simulink model "Fixed_Formation"  (R2014a)
settings: Solver=ode45  StartTime=0.0  StopTime=100.0  RelTol=1e-3
libraries: simulink x4
settings Model: Creator=asus  LastModifiedBy=asus

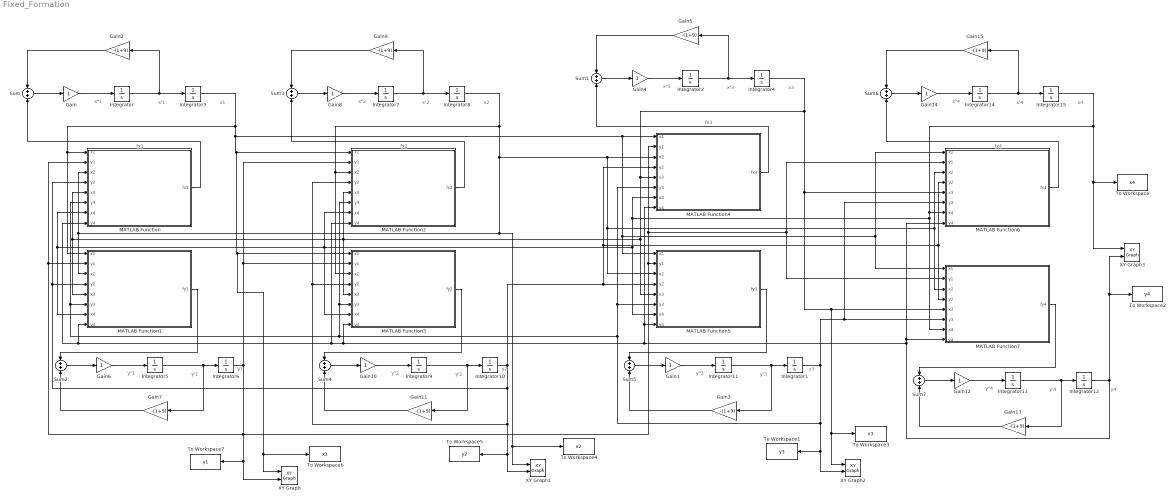
== system Fixed_Formation ==
  note: x1
  note: x'1
  note: x"1
  note: fx1
  note: y1
  note: y'1
  note: y"1
  note: x2
  note: x'2
  note: x"2
  note: fx2
  note: y2
  note: y'2
  note: y"2
  note: x3
  note: x'3
  note: x"3
  note: fx3
  note: y3
  note: y'3
  note: y"3
  note: x4
  note: x'4
  note: x"4
  note: fx4
  note: y4
  note: y'4
  note: y"4
  Gain{,1,4,6,8,10,12,14} (8 alike) : Gain
  Gain{2..3,5,7,9,11,13,15} (8 alike) : Gain  Gain=-(1+9)
  Integrator{,2,5,7,9,11,13..14} (8 alike) : Integrator
  Integrator1 : Integrator  InitialCondition=2
  Integrator10 : Integrator  InitialCondition=1
  Integrator12 : Integrator  InitialCondition=4
  Integrator15 : Integrator  InitialCondition=4
  Integrator3 : Integrator  InitialCondition=-3
  Integrator4 : Integrator  InitialCondition=5
  Integrator6 : Integrator  InitialCondition=3
  Integrator8 : Integrator  InitialCondition=1
  MATLAB Function : MATLAB Function  TreatAsAtomicUnit=on
  MATLAB Function1 : MATLAB Function  TreatAsAtomicUnit=on
  MATLAB Function2 : MATLAB Function  TreatAsAtomicUnit=on
  MATLAB Function3 : MATLAB Function  TreatAsAtomicUnit=on
  MATLAB Function4 : MATLAB Function  TreatAsAtomicUnit=on
  MATLAB Function5 : MATLAB Function  TreatAsAtomicUnit=on
  MATLAB Function6 : MATLAB Function  TreatAsAtomicUnit=on
  MATLAB Function7 : MATLAB Function  TreatAsAtomicUnit=on
  Sum{,1..7} (8 alike) : Sum  Inputs=+|+
  To Workspace : ToWorkspace  VariableName=x4  SampleTime=0.01
  To Workspace1 : ToWorkspace  VariableName=y3  SampleTime=0.01
  To Workspace2 : ToWorkspace  VariableName=y4  SampleTime=0.01
  To Workspace3 : ToWorkspace  VariableName=x3  SampleTime=0.01
  To Workspace4 : ToWorkspace  VariableName=x2  SampleTime=0.01
  To Workspace5 : ToWorkspace  VariableName=y2  SampleTime=0.01
  To Workspace6 : ToWorkspace  VariableName=x1  SampleTime=0.01
  To Workspace7 : ToWorkspace  VariableName=y1  SampleTime=0.01
  XY Graph{,1..3} (4 alike) : simulink/Sinks/XY Graph  xmin=-10  xmax=10  ymin=-10  ymax=10  st=0.01
  wires:
  Sum/1 -> Gain/1
  Gain/1 -> Integrator/1
  Integrator/1 -> Gain2/1, Integrator3/1
  Gain2/1 -> Sum/1
  Integrator3/1 -> MATLAB Function6/1(x1), MATLAB Function7/1(x1), MATLAB Function5/1(x1), MATLAB Function4/1(x1), To Workspace6/1, XY Graph/1, MATLAB Function3/1(x1), MATLAB Function2/1(x1), MATLAB Function/1(x1), MATLAB Function1/1(x1)
  Sum2/1 -> Gain6/1
  Gain6/1 -> Integrator5/1
  Integrator5/1 -> Gain7/1, Integrator6/1
  Gain7/1 -> Sum2/2
  MATLAB Function1/1(fy1) -> Sum2/1
  Sum3/1 -> Gain8/1
  Gain8/1 -> Integrator7/1
  Integrator7/1 -> Gain9/1, Integrator8/1
  Gain9/1 -> Sum3/1
  Integrator8/1 -> MATLAB Function7/3(x2), MATLAB Function6/3(x2), MATLAB Function5/3(x2), MATLAB Function4/3(x2), To Workspace4/1, XY Graph1/1, MATLAB Function1/3(x2), MATLAB Function/3(x2), MATLAB Function3/3(x2), MATLAB Function2/3(x2)
  MATLAB Function2/1(fx2) -> Sum3/2
  Sum4/1 -> Gain10/1
  Gain10/1 -> Integrator9/1
  Integrator9/1 -> Gain11/1, Integrator10/1
  Gain11/1 -> Sum4/2
  MATLAB Function3/1(fy2) -> Sum4/1
  Sum1/1 -> Gain4/1
  Gain4/1 -> Integrator2/1
  Integrator2/1 -> Gain5/1, Integrator4/1
  Gain5/1 -> Sum1/1
  MATLAB Function4/1(fx3) -> Sum1/2
  Sum5/1 -> Gain1/1
  Gain1/1 -> Integrator11/1
  Integrator11/1 -> Gain3/1, Integrator1/1
  Gain3/1 -> Sum5/2
  MATLAB Function5/1(fy3) -> Sum5/1
  Integrator1/1 -> MATLAB Function6/6(y3), MATLAB Function7/6(y3), To Workspace1/1, XY Graph2/2, MATLAB Function/6(y3), MATLAB Function1/6(y3), MATLAB Function3/6(y3), MATLAB Function2/6(y3), MATLAB Function5/6(y3), MATLAB Function4/6(y3)
  Sum6/1 -> Gain14/1
  Gain14/1 -> Integrator14/1
  Integrator14/1 -> Gain15/1, Integrator15/1
  Gain15/1 -> Sum6/1
  Integrator15/1 -> To Workspace/1, XY Graph3/1, MATLAB Function1/7(x4), MATLAB Function/7(x4), MATLAB Function3/7(x4), MATLAB Function2/7(x4), MATLAB Function5/7(x4), MATLAB Function4/7(x4), MATLAB Function7/7(x4), MATLAB Function6/7(x4)
  MATLAB Function6/1(fx4) -> Sum6/2
  Sum7/1 -> Gain12/1
  Gain12/1 -> Integrator13/1
  Integrator13/1 -> Gain13/1, Integrator12/1
  Gain13/1 -> Sum7/2
  MATLAB Function7/1(fy4) -> Sum7/1
  Integrator4/1 -> MATLAB Function6/5(x3), To Workspace3/1, XY Graph2/1, MATLAB Function7/5(x3), MATLAB Function4/5(x3), MATLAB Function5/5(x3), MATLAB Function1/5(x3), MATLAB Function/5(x3), MATLAB Function2/5(x3), MATLAB Function3/5(x3)
  Integrator12/1 -> To Workspace2/1, XY Graph3/2, MATLAB Function6/8(y4), MATLAB Function7/8(y4), MATLAB Function4/8(y4), MATLAB Function5/8(y4), MATLAB Function2/8(y4), MATLAB Function/8(y4), MATLAB Function1/8(y4), MATLAB Function3/8(y4)
  Integrator10/1 -> MATLAB Function6/4(y2), MATLAB Function7/4(y2), MATLAB Function4/4(y2), MATLAB Function5/4(y2), MATLAB Function/4(y2), MATLAB Function1/4(y2), To Workspace5/1, XY Graph1/2, MATLAB Function2/4(y2), MATLAB Function3/4(y2)
  Integrator6/1 -> MATLAB Function2/2(y1), MATLAB Function3/2(y1), To Workspace7/1, XY Graph/2, MATLAB Function7/2(y1), MATLAB Function6/2(y1), MATLAB Function4/2(y1), MATLAB Function5/2(y1), MATLAB Function/2(y1), MATLAB Function1/2(y1)
  MATLAB Function/1(fx1) -> Sum/2

== matlab function Fixed_Formation/MATLAB Function1 ==
  data: fy1 output; x1 input; y1 input; x2 input; y2 input; x3 input; y3 input; x4 input; y4 input
function fy1 = fy1(x1,y1,x2,y2,x3,y3,x4,y4)
%#codegen
% Agent N#1
%xc = sin(t);
%yc = t;

xc = 0;             % X-Center.
yc = 0;             % Y-Center.
al = 3;             % Radius.
x = [x1 x2 x3 x4];      
y = [y1 y2 y3 y4];     
M = 1;              % Mass.
B = 1;              % Damper.
kd = 9;             % Overshoot Controlling Coefficient.
ks = 1;
q = 10;     % Charges.
kr = 0.15;
N = 4;              % Number od Agents.

r2 = zeros(N,N);
costet = zeros(N,N);
sintet = zeros(N,N);
Prx = zeros(N);
Pry = zeros(N);

fx = zeros(N);
fy = zeros(N);
Fx = zeros(N);
Fy = zeros(N);

for k=1:N
    
    for i=1:N
      Pr = 0;
      r2(k,i) = ((x(i)-x(k))^2)+((y(i)-y(k))^2);
    
      if i==k
         Prx(k) = Prx(k) + 0;
         Pry(k) = Pry(k) + 0;
      else
         costet(k,i) = (x(k)-x(i))/sqrt(r2(k,i));
         sintet(k,i) = (y(k)-y(i))/sqrt(r2(k,i));
         Prx(k) = Prx(k) + (q*q/r2(k,i))*costet(k,i);
         Pry(k) = Pry(k) + (q*q/r2(k,i))*sintet(k,i);
        
      end
    end

    Fx(k) = kr*Prx(k);
    Fy(k) = kr*Pry(k);
                        
    fx(k) = Fx(k)-ks*((x(k)-xc)*(((x(k)-xc)^2)+((y(k)-yc)^2)-al^2));
    fy(k) = Fy(k)-ks*((y(k)-yc)*(((x(k)-xc)^2)+((y(k)-yc)^2)-al^2));

end

fy1 = fy(1);

end

== matlab function Fixed_Formation/MATLAB Function ==
  data: fx1 output; x1 input; y1 input; x2 input; y2 input; x3 input; y3 input; x4 input; y4 input
function fx1 = fx1(x1,y1,x2,y2,x3,y3,x4,y4)
%#codegen
% Agent N#1

xc = 0;             % X-Center.
yc = 0;             % Y-Center.
al = 3;             % Radius.
x = [x1 x2 x3 x4];      
y = [y1 y2 y3 y4];     
M = 1;              % Mass.
B = 1;              % Damper.
kd = 9;             % Overshoot Controlling Coefficient.
ks = 1;
q = 10;     % Charges.
kr = 0.15;
N = 4;              % Number od Agents.

r2 = zeros(N,N);
costet = zeros(N,N);
sintet = zeros(N,N);
Prx = zeros(N);
Pry = zeros(N);

fx = zeros(N);
fy = zeros(N);
Fx = zeros(N);
Fy = zeros(N);

for k=1:N
    
    for i=1:N
      Pr = 0;
      r2(k,i) = ((x(i)-x(k))^2)+((y(i)-y(k))^2);
    
      if i==k
         Prx(k) = Prx(k) + 0;
         Pry(k) = Pry(k) + 0;
      else
         costet(k,i) = (x(k)-x(i))/sqrt(r2(k,i));
         sintet(k,i) = (y(k)-y(i))/sqrt(r2(k,i));
         Prx(k) = Prx(k) + (q*q/r2(k,i))*costet(k,i);
         Pry(k) = Pry(k) + (q*q/r2(k,i))*sintet(k,i);
        
      end
    end

    Fx(k) = kr*Prx(k);
    Fy(k) = kr*Pry(k);
                        
    fx(k) = Fx(k)-ks*((x(k)-xc)*(((x(k)-xc)^2)+((y(k)-yc)^2)-al^2));
    fy(k) = Fy(k)-ks*((y(k)-yc)*(((x(k)-xc)^2)+((y(k)-yc)^2)-al^2));

end

fx1 = fx(1);

end

== matlab function Fixed_Formation/MATLAB Function2 ==
  data: fx2 output; x1 input; y1 input; x2 input; y2 input; x3 input; y3 input; x4 input; y4 input
function fx2 = fx2(x1,y1,x2,y2,x3,y3,x4,y4)
%#codegen
% Agent N#1

xc = 0;             % X-Center.
yc = 0;             % Y-Center.
al = 3;             % Radius.
x = [x1 x2 x3 x4];      
y = [y1 y2 y3 y4];     
M = 1;              % Mass.
B = 1;              % Damper.
kd = 9;             % Overshoot Controlling Coefficient.
ks = 1;
q = 10;     % Charges.
kr = 0.15;
N = 4;              % Number od Agents.

r2 = zeros(N,N);
costet = zeros(N,N);
sintet = zeros(N,N);
Prx = zeros(N);
Pry = zeros(N);

fx = zeros(N);
fy = zeros(N);
Fx = zeros(N);
Fy = zeros(N);

for k=1:N
    
    for i=1:N
      Pr = 0;
      r2(k,i) = ((x(i)-x(k))^2)+((y(i)-y(k))^2);
    
      if i==k
         Prx(k) = Prx(k) + 0;
         Pry(k) = Pry(k) + 0;
      else
         costet(k,i) = (x(k)-x(i))/sqrt(r2(k,i));
         sintet(k,i) = (y(k)-y(i))/sqrt(r2(k,i));
         Prx(k) = Prx(k) + (q*q/r2(k,i))*costet(k,i);
         Pry(k) = Pry(k) + (q*q/r2(k,i))*sintet(k,i);
        
      end
    end

    Fx(k) = kr*Prx(k);
    Fy(k) = kr*Pry(k);
                        
    fx(k) = Fx(k)-ks*((x(k)-xc)*(((x(k)-xc)^2)+((y(k)-yc)^2)-al^2));
    fy(k) = Fy(k)-ks*((y(k)-yc)*(((x(k)-xc)^2)+((y(k)-yc)^2)-al^2));

end

fx2 = fx(2);


end

== matlab function Fixed_Formation/MATLAB Function3 ==
  data: fy2 output; x1 input; y1 input; x2 input; y2 input; x3 input; y3 input; x4 input; y4 input
function fy2 = fy2(x1,y1,x2,y2,x3,y3,x4,y4)
%#codegen
% Agent N#1

xc = 0;             % X-Center.
yc = 0;             % Y-Center.
al = 3;             % Radius.
x = [x1 x2 x3 x4];      
y = [y1 y2 y3 y4];     
M = 1;              % Mass.
B = 1;              % Damper.
kd = 9;             % Overshoot Controlling Coefficient.
ks = 1;
q = 10;     % Charges.
kr = 0.15;
N = 4;              % Number od Agents.

r2 = zeros(N,N);
costet = zeros(N,N);
sintet = zeros(N,N);
Prx = zeros(N);
Pry = zeros(N);

fx = zeros(N);
fy = zeros(N);
Fx = zeros(N);
Fy = zeros(N);

for k=1:N
    
    for i=1:N
      Pr = 0;
      r2(k,i) = ((x(i)-x(k))^2)+((y(i)-y(k))^2);
    
      if i==k
         Prx(k) = Prx(k) + 0;
         Pry(k) = Pry(k) + 0;
      else
         costet(k,i) = (x(k)-x(i))/sqrt(r2(k,i));
         sintet(k,i) = (y(k)-y(i))/sqrt(r2(k,i));
         Prx(k) = Prx(k) + (q*q/r2(k,i))*costet(k,i);
         Pry(k) = Pry(k) + (q*q/r2(k,i))*sintet(k,i);
        
      end
    end

    Fx(k) = kr*Prx(k);
    Fy(k) = kr*Pry(k);
                        
    fx(k) = Fx(k)-ks*((x(k)-xc)*(((x(k)-xc)^2)+((y(k)-yc)^2)-al^2));
    fy(k) = Fy(k)-ks*((y(k)-yc)*(((x(k)-xc)^2)+((y(k)-yc)^2)-al^2));

end

fy2 = fy(2);


end

== matlab function Fixed_Formation/MATLAB Function4 ==
  data: fx3 output; x1 input; y1 input; x2 input; y2 input; x3 input; y3 input; x4 input; y4 input
function fx3 = fx3(x1,y1,x2,y2,x3,y3,x4,y4)
%#codegen
% Agent N#1

xc = 0;             % X-Center.
yc = 0;             % Y-Center.
al = 3;             % Radius.
x = [x1 x2 x3 x4];      
y = [y1 y2 y3 y4];     
M = 1;              % Mass.
B = 1;              % Damper.
kd = 9;             % Overshoot Controlling Coefficient.
ks = 1;
q = 10;     % Charges.
kr = 0.15;
N = 4;              % Number od Agents.

r2 = zeros(N,N);
costet = zeros(N,N);
sintet = zeros(N,N);
Prx = zeros(N);
Pry = zeros(N);

fx = zeros(N);
fy = zeros(N);
Fx = zeros(N);
Fy = zeros(N);

for k=1:N
    
    for i=1:N
      Pr = 0;
      r2(k,i) = ((x(i)-x(k))^2)+((y(i)-y(k))^2);
    
      if i==k
         Prx(k) = Prx(k) + 0;
         Pry(k) = Pry(k) + 0;
      else
         costet(k,i) = (x(k)-x(i))/sqrt(r2(k,i));
         sintet(k,i) = (y(k)-y(i))/sqrt(r2(k,i));
         Prx(k) = Prx(k) + (q*q/r2(k,i))*costet(k,i);
         Pry(k) = Pry(k) + (q*q/r2(k,i))*sintet(k,i);
        
      end
    end

    Fx(k) = kr*Prx(k);
    Fy(k) = kr*Pry(k);
                        
    fx(k) = Fx(k)-ks*((x(k)-xc)*(((x(k)-xc)^2)+((y(k)-yc)^2)-al^2));
    fy(k) = Fy(k)-ks*((y(k)-yc)*(((x(k)-xc)^2)+((y(k)-yc)^2)-al^2));

end

fx3 = fx(3);


end

== matlab function Fixed_Formation/MATLAB Function5 ==
  data: fy3 output; x1 input; y1 input; x2 input; y2 input; x3 input; y3 input; x4 input; y4 input
function fy3 = fy3(x1,y1,x2,y2,x3,y3,x4,y4)
%#codegen
% Agent N#1

xc = 0;             % X-Center.
yc = 0;             % Y-Center.
al = 3;             % Radius.
x = [x1 x2 x3 x4];      
y = [y1 y2 y3 y4];     
M = 1;              % Mass.
B = 1;              % Damper.
kd = 9;             % Overshoot Controlling Coefficient.
ks = 1;
q = 10;     % Charges.
kr = 0.15;
N = 4;              % Number od Agents.

r2 = zeros(N,N);
costet = zeros(N,N);
sintet = zeros(N,N);
Prx = zeros(N);
Pry = zeros(N);

fx = zeros(N);
fy = zeros(N);
Fx = zeros(N);
Fy = zeros(N);

for k=1:N
    
    for i=1:N
      Pr = 0;
      r2(k,i) = ((x(i)-x(k))^2)+((y(i)-y(k))^2);
    
      if i==k
         Prx(k) = Prx(k) + 0;
         Pry(k) = Pry(k) + 0;
      else
         costet(k,i) = (x(k)-x(i))/sqrt(r2(k,i));
         sintet(k,i) = (y(k)-y(i))/sqrt(r2(k,i));
         Prx(k) = Prx(k) + (q*q/r2(k,i))*costet(k,i);
         Pry(k) = Pry(k) + (q*q/r2(k,i))*sintet(k,i);
        
      end
    end

    Fx(k) = kr*Prx(k);
    Fy(k) = kr*Pry(k);
                        
    fx(k) = Fx(k)-ks*((x(k)-xc)*(((x(k)-xc)^2)+((y(k)-yc)^2)-al^2));
    fy(k) = Fy(k)-ks*((y(k)-yc)*(((x(k)-xc)^2)+((y(k)-yc)^2)-al^2));

end

fy3 = fy(3);


end

== matlab function Fixed_Formation/MATLAB Function6 ==
  data: fx4 output; x1 input; y1 input; x2 input; y2 input; x3 input; y3 input; x4 input; y4 input
function fx4 = fx4(x1,y1,x2,y2,x3,y3,x4,y4)
%#codegen
% Agent N#1

xc = 0;             % X-Center.
yc = 0;             % Y-Center.
al = 3;             % Radius.
x = [x1 x2 x3 x4];      
y = [y1 y2 y3 y4];     
M = 1;              % Mass.
B = 1;              % Damper.
kd = 9;             % Overshoot Controlling Coefficient.
ks = 1;
q = 10;     % Charges.
kr = 0.15;
N = 4;              % Number od Agents.

r2 = zeros(N,N);
costet = zeros(N,N);
sintet = zeros(N,N);
Prx = zeros(N);
Pry = zeros(N);

fx = zeros(N);
fy = zeros(N);
Fx = zeros(N);
Fy = zeros(N);

for k=1:N
    
    for i=1:N
      Pr = 0;
      r2(k,i) = ((x(i)-x(k))^2)+((y(i)-y(k))^2);
    
      if i==k
         Prx(k) = Prx(k) + 0;
         Pry(k) = Pry(k) + 0;
      else
         costet(k,i) = (x(k)-x(i))/sqrt(r2(k,i));
         sintet(k,i) = (y(k)-y(i))/sqrt(r2(k,i));
         Prx(k) = Prx(k) + (q*q/r2(k,i))*costet(k,i);
         Pry(k) = Pry(k) + (q*q/r2(k,i))*sintet(k,i);
        
      end
    end

    Fx(k) = kr*Prx(k);
    Fy(k) = kr*Pry(k);
                        
    fx(k) = Fx(k)-ks*((x(k)-xc)*(((x(k)-xc)^2)+((y(k)-yc)^2)-al^2));
    fy(k) = Fy(k)-ks*((y(k)-yc)*(((x(k)-xc)^2)+((y(k)-yc)^2)-al^2));

end

fx4 = fx(4);


end

== matlab function Fixed_Formation/MATLAB Function7 ==
  data: fy4 output; x1 input; y1 input; x2 input; y2 input; x3 input; y3 input; x4 input; y4 input
function fy4 = fy4(x1,y1,x2,y2,x3,y3,x4,y4)
%#codegen
% Agent N#1

xc = 0;             % X-Center.
yc = 0;             % Y-Center.
al = 3;             % Radius.
x = [x1 x2 x3 x4];      
y = [y1 y2 y3 y4];     
M = 1;              % Mass.
B = 1;              % Damper.
kd = 9;             % Overshoot Controlling Coefficient.
ks = 1;
q = 10;     % Charges.
kr = 0.15;
N = 4;              % Number od Agents.

r2 = zeros(N,N);
costet = zeros(N,N);
sintet = zeros(N,N);
Prx = zeros(N);
Pry = zeros(N);

fx = zeros(N);
fy = zeros(N);
Fx = zeros(N);
Fy = zeros(N);

for k=1:N
    
    for i=1:N
      Pr = 0;
      r2(k,i) = ((x(i)-x(k))^2)+((y(i)-y(k))^2);
    
      if i==k
         Prx(k) = Prx(k) + 0;
         Pry(k) = Pry(k) + 0;
      else
         costet(k,i) = (x(k)-x(i))/sqrt(r2(k,i));
         sintet(k,i) = (y(k)-y(i))/sqrt(r2(k,i));
         Prx(k) = Prx(k) + (q*q/r2(k,i))*costet(k,i);
         Pry(k) = Pry(k) + (q*q/r2(k,i))*sintet(k,i);
        
      end
    end

    Fx(k) = kr*Prx(k);
    Fy(k) = kr*Pry(k);
                        
    fx(k) = Fx(k)-ks*((x(k)-xc)*(((x(k)-xc)^2)+((y(k)-yc)^2)-al^2));
    fy(k) = Fy(k)-ks*((y(k)-yc)*(((x(k)-xc)^2)+((y(k)-yc)^2)-al^2));

end

fy4 = fy(4);


end
